simulink model "simu_complete_ASMC"  (R2024b)
settings: Solver=FixedStepAuto  StartTime=0.0  StopTime=Tsim  FixedStep=Ts  RelTol=1e-3
values from neighbouring files (symbols this model uses):
  delta0 = 10    [getItRunning.m]
  deltaF = -10    [getItRunning.m]
  Re = 0.228    [main_data_vehicle.m]
  t_sw = 5    [getItRunning.m]
  Tr = 0.2    [getItRunning.m]
  v0 = 10    [getItRunning.m]    (also in main_data_vehicle.m = 1)
settings Model: Creator=marti  LastModifiedBy=Filip

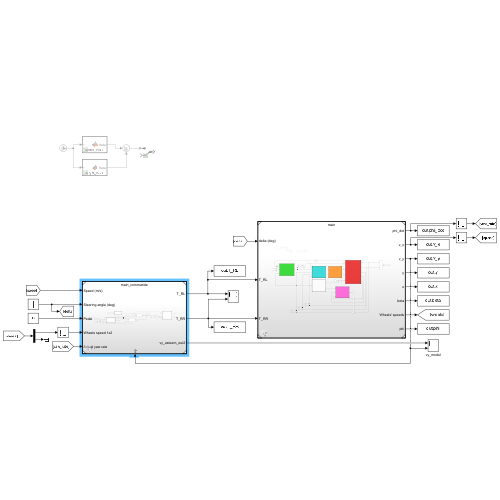
[thumbnail: Simulink's stored preview of the top-level diagram]
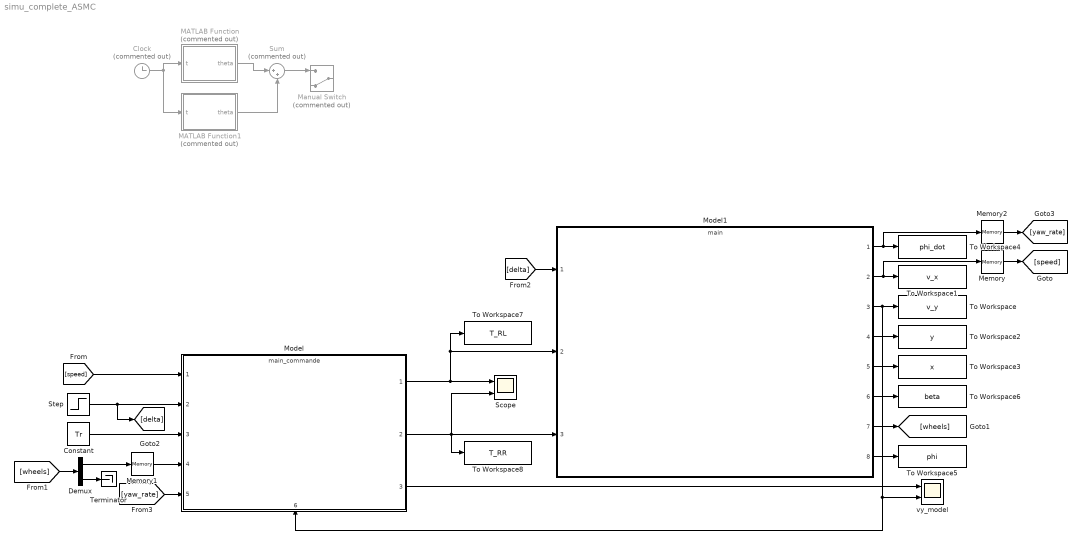
== system simu_complete_ASMC ==
  Clock : Clock  Commented=on
  Constant : Constant  Value=Tr
  Demux : Demux  Outputs=2
  MATLAB Function : MATLAB Function  Commented=on  TreatAsAtomicUnit=on
  MATLAB Function1 : MATLAB Function  Commented=on  TreatAsAtomicUnit=on
  Manual Switch : ManualSwitch  Commented=on  CurrentSetting=0
  Memory : Memory  InitialCondition=v0
  Memory1 : Memory  InitialCondition=[v0/Re v0/Re]
  Memory2 : Memory
  Model : ModelReference  ModelNameDialog=main_commande.slx  SimulationMode=Normal  ModelReferenceVersion=1.47
      settings: PortSchema="{\"entries\":[{\"content\":{\"sides\":[{\"content\":{\"connectorIds\":[\"In1\",\"In2\",\"In3\",\"In4\",\"In5\"]},\"type\":\"ConnectorPlacement.EquallySpacedRectSide\",\"uuid\":\"422f371f-fcb3-40d1-9c6b-2b45da2fc934\"},{\"content\":{\"connectorIds\":[\"Out1\",\"Out2\",\"Out3\"],\"side\":\"RIGHT\"},\"type\":\"ConnectorPlacement.EquallySpacedRectSide\",\"uuid\":\"5fd8a801-8d83-4f2f-88b4-f69183b19fb5\"},{\"content\":{\"side\":\"TOP\"},\"type\":\"ConnectorPlacement.EquallySpacedRectSide\",\"uuid\":\"80dd5862-0201-4630-9f15-61d2f39f9c33\"},{\"content\":{\"connectorIds\":[\"In6\"],\"side\":\"BOTTOM\"},\"type\":\"ConnectorPlacement.EquallySpacedRectSide\",\"uuid\":\"ea91b8b9-3e6a-4d71-9b35-4e9622753c2b\"}]},\"type\":\"ConnectorPlacement.EquallySpacedConnector\",\"uuid\":\"5526fd4a-c22c-4e82-871e-4b54d21dd880\"}],\"packageUris\":[\"http://schema.mathworks.com/mf0/Connector/R2020b\"],\"version\":\"1.0\"}"
  Model1 : ModelReference  ModelNameDialog=main.slx  SimulationMode=Normal  ModelReferenceVersion=1.137
  Scope : Scope  NumInputPorts=2
  Step : Step  Time=t_sw  Before=delta0  After=deltaF  SampleTime=0
  Sum : Sum  Commented=on  Inputs=|++
  Terminator : Terminator
  To Workspace : ToWorkspace  VariableName=v_y  SaveFormat=Structure With Time  SampleTime=-1
  To Workspace1 : ToWorkspace  VariableName=v_x  SaveFormat=Structure With Time  SampleTime=-1
  To Workspace2 : ToWorkspace  VariableName=y  SaveFormat=Structure With Time  SampleTime=-1
  To Workspace3 : ToWorkspace  VariableName=x  SaveFormat=Structure With Time  SampleTime=-1
  To Workspace4 : ToWorkspace  VariableName=phi_dot  SaveFormat=Structure With Time  SampleTime=-1
  To Workspace5 : ToWorkspace  VariableName=phi  SaveFormat=Structure With Time  SampleTime=-1
  To Workspace6 : ToWorkspace  VariableName=beta  SaveFormat=Structure With Time  SampleTime=-1
  To Workspace7 : ToWorkspace  VariableName=T_RL  SaveFormat=Structure With Time  SampleTime=-1
  To Workspace8 : ToWorkspace  VariableName=T_RR  SaveFormat=Structure With Time  SampleTime=-1
  vy_model : Scope  NumInputPorts=2
  wires:
  Model1/2 -> To Workspace1/1, Memory/1
  [speed] -> Model/1
  [wheels] -> Demux/1
  Demux/1 -> Memory1/1
  Clock/1 -> MATLAB Function1/1(t), MATLAB Function/1(t)
  Constant/1 -> Model/3
  [delta] -> Model1/1
  Memory/1 -> [speed]
  Model1/7 -> [wheels]
  Memory1/1 -> Model/4
  Model1/1 -> To Workspace4/1, Memory2/1
  Memory2/1 -> [yaw_rate]
  Sum/1 -> Manual Switch/1
  Step/1 -> [delta], Model/2
  [yaw_rate] -> Model/5
  MATLAB Function/1(theta) -> Sum/1
  MATLAB Function1/1(theta) -> Sum/2
  Demux/2 -> Terminator/1
  Model1/8 -> To Workspace5/1
  Model1/4 -> To Workspace2/1
  Model1/5 -> To Workspace3/1
  Model1/6 -> To Workspace6/1
  Model/1 -> Scope/1, Model1/2, To Workspace7/1
  Model/2 -> To Workspace8/1, Scope/2, Model1/3
  Model/3 -> vy_model/1
  Model1/3 -> Model/6, vy_model/2, To Workspace/1

== matlab function simu_complete_ASMC/MATLAB Function ==
  data: t input; theta output
function theta = angle_roue(t)
    % Fonction pour modéliser l'angle de roue d'un double changement de voie
    % Entrée :
    %   t : vecteur ou scalaire temps
    % Sortie :
    %   theta : angle de roue correspondant à chaque t

    theta = zeros(size(t));  % Initialisation

    % Intervalle actif : [1,4]
    idx = (t > 1) & (t < 4);
    
    % Fonction sinus entre 2 et 5 (période complète sur 3 secondes)
    theta(idx) = sin(2*pi * (t(idx) - 1) / 3);
end

== matlab function simu_complete_ASMC/MATLAB Function1 ==
  data: t input; theta output
function theta = angle_roue(t)
    % Fonction pour modéliser l'angle de roue d'un double changement de voie
    % Entrée :
    %   t : vecteur ou scalaire temps
    % Sortie :
    %   theta : angle de roue correspondant à chaque t

    theta = zeros(size(t));  % Initialisation

    % Intervalle actif : [5,8]
    idx = (t > 6) & (t < 9);
    
    % Fonction sinus entre 2 et 5 (période complète sur 3 secondes)
    theta(idx) = -sin(2*pi * (t(idx) - 6) / 3);
end
